simulink model "DDMR_sim_imputW"  (R2022a)
settings: Solver=FixedStepAuto  StartTime=0.0  StopTime=10.0  FixedStep=0.001  RelTol=1e-3
values from neighbouring files (symbols this model uses):
  Cm = 0    [DDMR_sim_imputW_set.m]
  Jm = 15.5*10^-7    (= 1.55e-06)    [DDMR_sim_imputW_set.m]
  Kb = Kt    (= 0.0286)    [DDMR_sim_imputW_set.m]
  Kf = 0    [DDMR_sim_imputW_set.m]
  Kt = 28.6*10^-3    (= 0.0286)    [DDMR_sim_imputW_set.m]
  La = 0.39*10^-3    (= 0.00039)    [DDMR_sim_imputW_set.m]
  N = N_motor * N_wheel    (= 1400)    [DDMR_sim_imputW_set.m]
  Ra = 0.38    [DDMR_sim_imputW_set.m]
libraries: simulink x2
settings Model: Creator=CSPLAB  LastModifiedBy=CSPLAB
settings DataIOCC: ReturnWorkspaceOutputs=off

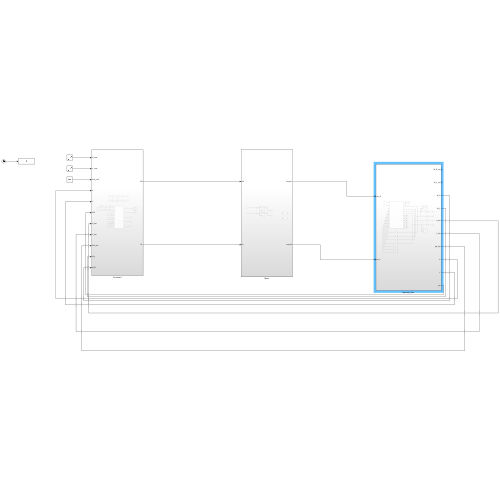
[thumbnail: Simulink's stored preview of the top-level diagram]
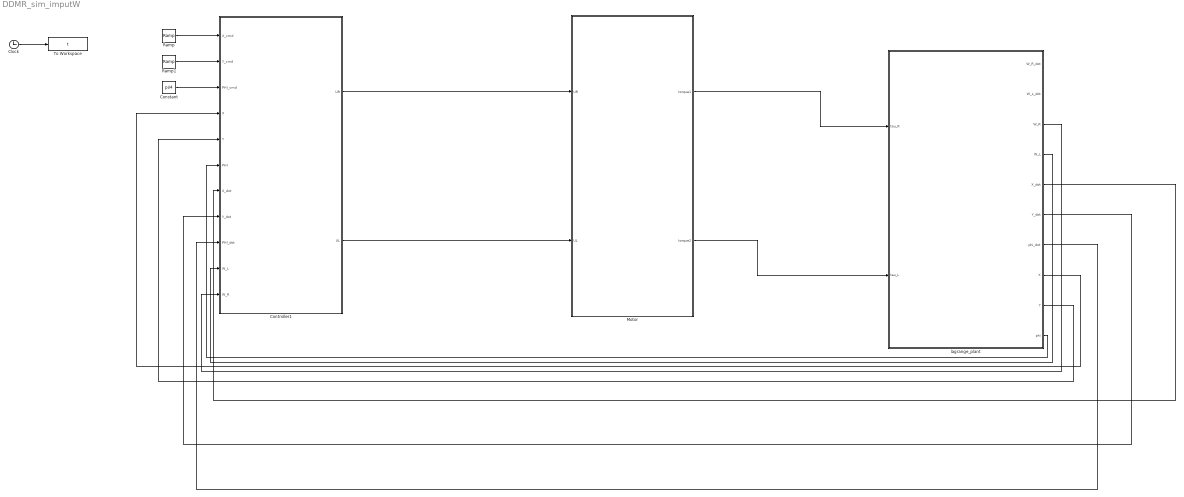
== system DDMR_sim_imputW ==
  Clock : Clock
  Constant : Constant  Value=pi/4
  Controller1 : Subsystem
  Motor : Subsystem
  Ramp : simulink/Sources/Ramp  slope=1  start=0  InitialOutput=0
  Ramp1 : simulink/Sources/Ramp  slope=1  start=0  InitialOutput=0
  To Workspace : ToWorkspace  VariableName=t  SaveFormat=Timeseries  SampleTime=-1
  lagrange_plant : Subsystem
  wires:
  Controller1/1(UR) -> Motor/1(UR)
  Controller1/2(UL) -> Motor/2(UL)
  Motor/1(torque1) -> lagrange_plant/1(tau_R)
  Motor/2(torque2) -> lagrange_plant/2(tau_L)
  lagrange_plant/3(W_R) -> Controller1/11(W_R)
  lagrange_plant/4(W_L) -> Controller1/10(W_L)
  Ramp1/1 -> Controller1/2(Y_cmd)
  Ramp/1 -> Controller1/1(X_cmd)
  Constant/1 -> Controller1/3(PHI_cmd)
  Clock/1 -> To Workspace/1
  lagrange_plant/10(phi) -> Controller1/6(PHI)
  lagrange_plant/5(X_dot) -> Controller1/7(X_dot)
  lagrange_plant/6(Y_dot) -> Controller1/8(Y_dot)
  lagrange_plant/7(phi_dot) -> Controller1/9(PHI_dot)
  lagrange_plant/8(X) -> Controller1/4(X)
  lagrange_plant/9(Y) -> Controller1/5(Y)

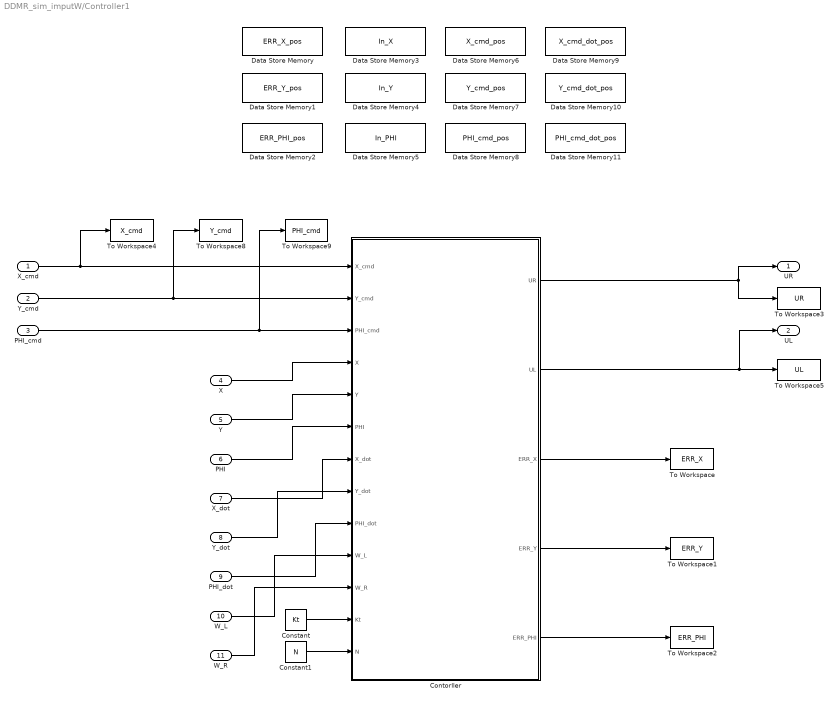
== system DDMR_sim_imputW/Controller1 ==
  X_cmd : Inport
  Y_cmd : Inport  Port=2
  PHI_cmd : Inport  Port=3
  X : Inport  Port=4
  Y : Inport  Port=5
  PHI : Inport  Port=6
  X_dot : Inport  Port=7
  Y_dot : Inport  Port=8
  PHI_dot : Inport  Port=9
  W_L : Inport  Port=10
  W_R : Inport  Port=11
  Constant : Constant  Value=Kt
  Constant1 : Constant  Value=N
  "Contorller " : MATLAB Function  TreatAsAtomicUnit=on
  Data Store Memory : DataStoreMemory  DataStoreName=ERR_X_pos  ReadBeforeWriteMsg=warning  WriteAfterWriteMsg=warning  WriteAfterReadMsg=warning  ShowAdditionalParam=off  OutDataTypeStr=double
  Data Store Memory1 : DataStoreMemory  DataStoreName=ERR_Y_pos  ReadBeforeWriteMsg=warning  WriteAfterWriteMsg=warning  WriteAfterReadMsg=warning  ShowAdditionalParam=off  OutDataTypeStr=double
  Data Store Memory10 : DataStoreMemory  DataStoreName=Y_cmd_dot_pos  ReadBeforeWriteMsg=warning  WriteAfterWriteMsg=warning  WriteAfterReadMsg=warning  ShowAdditionalParam=off  OutDataTypeStr=double
  Data Store Memory11 : DataStoreMemory  DataStoreName=PHI_cmd_dot_pos  ReadBeforeWriteMsg=warning  WriteAfterWriteMsg=warning  WriteAfterReadMsg=warning  ShowAdditionalParam=off  OutDataTypeStr=double
  Data Store Memory2 : DataStoreMemory  DataStoreName=ERR_PHI_pos  ReadBeforeWriteMsg=warning  WriteAfterWriteMsg=warning  WriteAfterReadMsg=warning  ShowAdditionalParam=off  OutDataTypeStr=double
  Data Store Memory3 : DataStoreMemory  DataStoreName=In_X  ReadBeforeWriteMsg=warning  WriteAfterWriteMsg=warning  WriteAfterReadMsg=warning  ShowAdditionalParam=off  OutDataTypeStr=double
  Data Store Memory4 : DataStoreMemory  DataStoreName=In_Y  ReadBeforeWriteMsg=warning  WriteAfterWriteMsg=warning  WriteAfterReadMsg=warning  ShowAdditionalParam=off  OutDataTypeStr=double
  Data Store Memory5 : DataStoreMemory  DataStoreName=In_PHI  ReadBeforeWriteMsg=warning  WriteAfterWriteMsg=warning  WriteAfterReadMsg=warning  ShowAdditionalParam=off  OutDataTypeStr=double
  Data Store Memory6 : DataStoreMemory  DataStoreName=X_cmd_pos  ReadBeforeWriteMsg=warning  WriteAfterWriteMsg=warning  WriteAfterReadMsg=warning  ShowAdditionalParam=off  OutDataTypeStr=double
  Data Store Memory7 : DataStoreMemory  DataStoreName=Y_cmd_pos  ReadBeforeWriteMsg=warning  WriteAfterWriteMsg=warning  WriteAfterReadMsg=warning  ShowAdditionalParam=off  OutDataTypeStr=double
  Data Store Memory8 : DataStoreMemory  DataStoreName=PHI_cmd_pos  ReadBeforeWriteMsg=warning  WriteAfterWriteMsg=warning  WriteAfterReadMsg=warning  ShowAdditionalParam=off  OutDataTypeStr=double
  Data Store Memory9 : DataStoreMemory  DataStoreName=X_cmd_dot_pos  ReadBeforeWriteMsg=warning  WriteAfterWriteMsg=warning  WriteAfterReadMsg=warning  ShowAdditionalParam=off  OutDataTypeStr=double
  To Workspace : ToWorkspace  VariableName=ERR_X  SampleTime=-1
  To Workspace1 : ToWorkspace  VariableName=ERR_Y  SampleTime=-1
  To Workspace2 : ToWorkspace  VariableName=ERR_PHI  SampleTime=-1
  To Workspace3 : ToWorkspace  VariableName=UR  SampleTime=-1
  To Workspace4 : ToWorkspace  VariableName=X_cmd  SampleTime=-1
  To Workspace5 : ToWorkspace  VariableName=UL  SampleTime=-1
  To Workspace8 : ToWorkspace  VariableName=Y_cmd  SampleTime=-1
  To Workspace9 : ToWorkspace  VariableName=PHI_cmd  SampleTime=-1
  UR : Outport  VectorParamsAs1DForOutWhenUnconnected=off
  UL : Outport  Port=2  VectorParamsAs1DForOutWhenUnconnected=off
  wires:
  "Contorller "/2(UL) -> UL/1, To Workspace5/1
  "Contorller "/1(UR) -> UR/1, To Workspace3/1
  W_R/1 -> "Contorller "/11(W_R)
  W_L/1 -> "Contorller "/10(W_L)
  PHI_dot/1 -> "Contorller "/9(PHI_dot)
  Y_dot/1 -> "Contorller "/8(Y_dot)
  X_dot/1 -> "Contorller "/7(X_dot)
  PHI/1 -> "Contorller "/6(PHI)
  Y/1 -> "Contorller "/5(Y)
  X/1 -> "Contorller "/4(X)
  PHI_cmd/1 -> To Workspace9/1, "Contorller "/3(PHI_cmd)
  Y_cmd/1 -> To Workspace8/1, "Contorller "/2(Y_cmd)
  X_cmd/1 -> To Workspace4/1, "Contorller "/1(X_cmd)
  Constant/1 -> "Contorller "/12(Kt)
  Constant1/1 -> "Contorller "/13(N)
  "Contorller "/5(ERR_PHI) -> To Workspace2/1
  "Contorller "/4(ERR_Y) -> To Workspace1/1
  "Contorller "/3(ERR_X) -> To Workspace/1

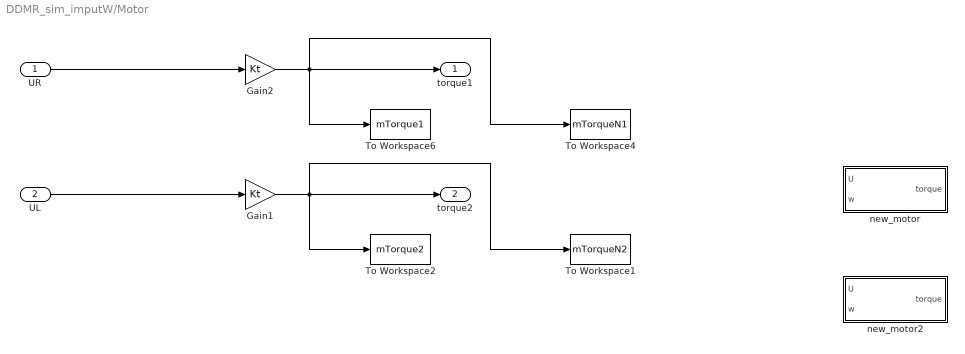
== system DDMR_sim_imputW/Motor ==
  UR : Inport
  UL : Inport  Port=2
  Gain1 : Gain  Gain=Kt
  Gain2 : Gain  Gain=Kt
  To Workspace1 : ToWorkspace  VariableName=mTorqueN2  SampleTime=-1
  To Workspace2 : ToWorkspace  VariableName=mTorque2  SampleTime=-1
  To Workspace4 : ToWorkspace  VariableName=mTorqueN1  SampleTime=-1
  To Workspace6 : ToWorkspace  VariableName=mTorque1  SampleTime=-1
  new_motor : Subsystem
  new_motor2 : Subsystem
  torque1 : Outport  VectorParamsAs1DForOutWhenUnconnected=off
  torque2 : Outport  Port=2  VectorParamsAs1DForOutWhenUnconnected=off
  wires:
  UR/1 -> Gain2/1
  Gain2/1 -> To Workspace6/1, To Workspace4/1, torque1/1
  Gain1/1 -> To Workspace2/1, To Workspace1/1, torque2/1
  UL/1 -> Gain1/1

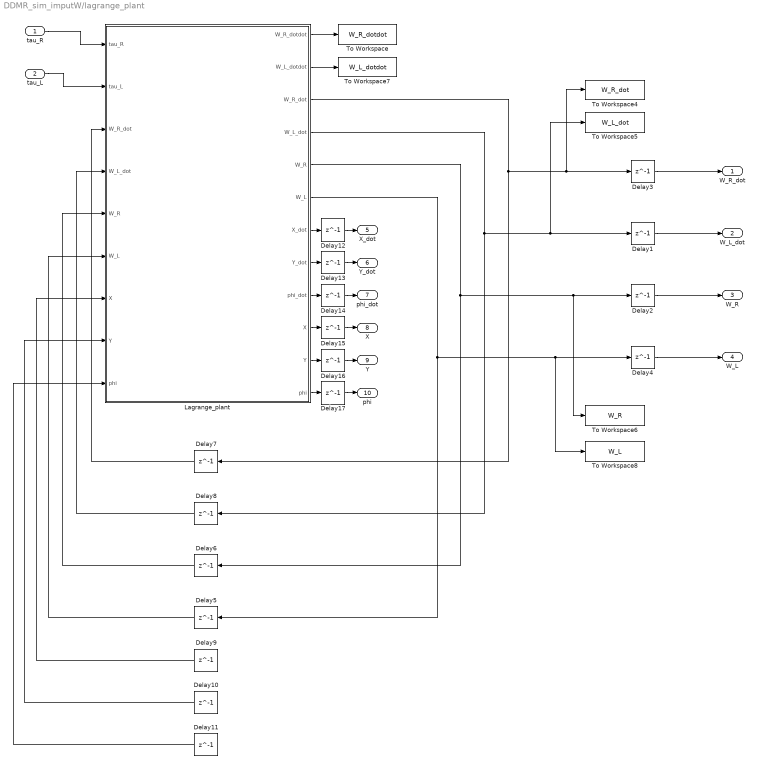
== system DDMR_sim_imputW/lagrange_plant ==
  tau_R : Inport
  tau_L : Inport  Port=2
  Delay{1..17} (17 alike) : Delay  DelayLength=1  InitialCondition=0
  Lagrange_plant : MATLAB Function  TreatAsAtomicUnit=on
  To Workspace : ToWorkspace  VariableName=W_R_dotdot  SaveFormat=Timeseries  SampleTime=-1
  To Workspace4 : ToWorkspace  VariableName=W_R_dot  SaveFormat=Timeseries  SampleTime=-1
  To Workspace5 : ToWorkspace  VariableName=W_L_dot  SaveFormat=Timeseries  SampleTime=-1
  To Workspace6 : ToWorkspace  VariableName=W_R  SaveFormat=Timeseries  SampleTime=-1
  To Workspace7 : ToWorkspace  VariableName=W_L_dotdot  SaveFormat=Timeseries  SampleTime=-1
  To Workspace8 : ToWorkspace  VariableName=W_L  SaveFormat=Timeseries  SampleTime=-1
  W_R_dot : Outport
  W_L_dot : Outport  Port=2
  W_R : Outport  Port=3
  W_L : Outport  Port=4
  X_dot : Outport  Port=5
  Y_dot : Outport  Port=6
  phi_dot : Outport  Port=7
  X : Outport  Port=8
  Y : Outport  Port=9
  phi : Outport  Port=10
  wires:
  Lagrange_plant/1(W_R_dotdot) -> To Workspace/1
  Lagrange_plant/2(W_L_dotdot) -> To Workspace7/1
  Delay1/1 -> W_L_dot/1
  Delay3/1 -> W_R_dot/1
  Delay2/1 -> W_R/1
  Delay4/1 -> W_L/1
  Lagrange_plant/6(W_L) -> Delay5/1, To Workspace8/1, Delay4/1
  Lagrange_plant/5(W_R) -> Delay6/1, To Workspace6/1, Delay2/1
  Lagrange_plant/4(W_L_dot) -> Delay8/1, Delay1/1, To Workspace5/1
  Lagrange_plant/3(W_R_dot) -> Delay7/1, To Workspace4/1, Delay3/1
  Delay7/1 -> Lagrange_plant/3("W_R_dot ")
  Delay8/1 -> Lagrange_plant/4("W_L_dot ")
  Delay6/1 -> Lagrange_plant/5("W_R ")
  Delay5/1 -> Lagrange_plant/6("W_L ")
  tau_R/1 -> Lagrange_plant/1(tau_R)
  tau_L/1 -> Lagrange_plant/2(tau_L)
  Delay9/1 -> Lagrange_plant/7("X ")
  Delay10/1 -> Lagrange_plant/8("Y ")
  Delay11/1 -> Lagrange_plant/9("phi ")
  Lagrange_plant/7(X_dot) -> Delay12/1
  Delay12/1 -> X_dot/1
  Lagrange_plant/8(Y_dot) -> Delay13/1
  Delay13/1 -> Y_dot/1
  Lagrange_plant/9(phi_dot) -> Delay14/1
  Delay14/1 -> phi_dot/1
  Lagrange_plant/10(X) -> Delay15/1
  Delay15/1 -> X/1
  Lagrange_plant/11(Y) -> Delay16/1
  Delay16/1 -> Y/1
  Lagrange_plant/12(phi) -> Delay17/1
  Delay17/1 -> phi/1

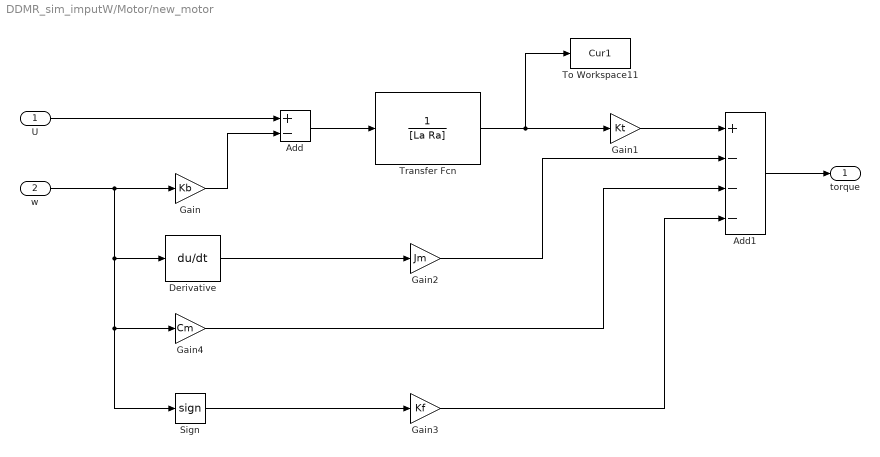
== system DDMR_sim_imputW/Motor/new_motor ==
  U : Inport
  w : Inport  Port=2
  Add : Sum  Inputs=+-
  Add1 : Sum  Inputs=+---
  Derivative : Derivative
  Gain : Gain  Gain=Kb
  Gain1 : Gain  Gain=Kt
  Gain2 : Gain  Gain=Jm
  Gain3 : Gain  Gain=Kf
  Gain4 : Gain  Gain=Cm
  Sign : Signum  ZeroCross=off
  To Workspace11 : ToWorkspace  VariableName=Cur1  SampleTime=-1
  Transfer Fcn : TransferFcn  Denominator=[La Ra]
  torque : Outport  VectorParamsAs1DForOutWhenUnconnected=off
  wires:
  Add1/1 -> torque/1
  Gain2/1 -> Add1/2
  Derivative/1 -> Gain2/1
  Gain1/1 -> Add1/1
  Gain4/1 -> Add1/3
  Gain/1 -> Add/2
  Transfer Fcn/1 -> To Workspace11/1, Gain1/1
  Sign/1 -> Gain3/1
  w/1 -> Sign/1, Gain4/1, Derivative/1, Gain/1
  U/1 -> Add/1
  Gain3/1 -> Add1/4
  Add/1 -> Transfer Fcn/1

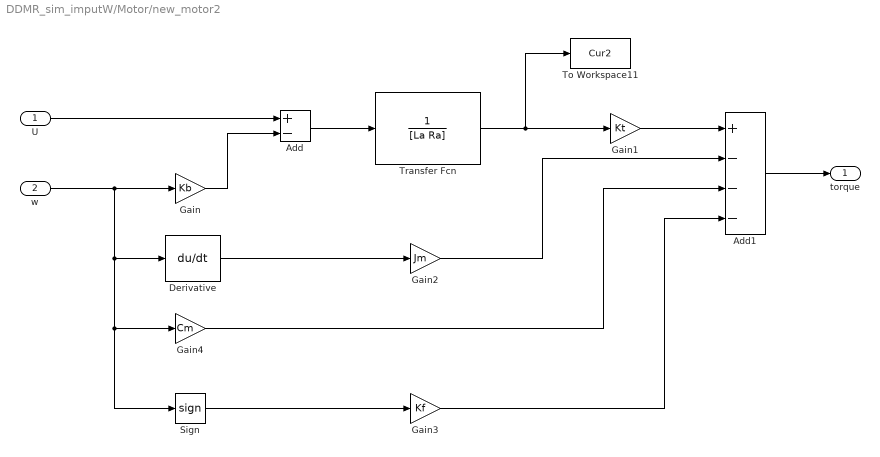
== system DDMR_sim_imputW/Motor/new_motor2 ==
  U : Inport
  w : Inport  Port=2
  Add : Sum  Inputs=+-
  Add1 : Sum  Inputs=+---
  Derivative : Derivative
  Gain : Gain  Gain=Kb
  Gain1 : Gain  Gain=Kt
  Gain2 : Gain  Gain=Jm
  Gain3 : Gain  Gain=Kf
  Gain4 : Gain  Gain=Cm
  Sign : Signum  ZeroCross=off
  To Workspace11 : ToWorkspace  VariableName=Cur2  SampleTime=-1
  Transfer Fcn : TransferFcn  Denominator=[La Ra]
  torque : Outport  VectorParamsAs1DForOutWhenUnconnected=off
  wires:
  Add1/1 -> torque/1
  Gain2/1 -> Add1/2
  Derivative/1 -> Gain2/1
  Gain1/1 -> Add1/1
  Gain4/1 -> Add1/3
  Add/1 -> Transfer Fcn/1
  Gain/1 -> Add/2
  Transfer Fcn/1 -> To Workspace11/1, Gain1/1
  Sign/1 -> Gain3/1
  w/1 -> Sign/1, Gain4/1, Derivative/1, Gain/1
  U/1 -> Add/1
  Gain3/1 -> Add1/4

== matlab function DDMR_sim_imputW/lagrange_plant/Lagrange_plant ==
  data: tau_R input; W_R_dotdot output; tau_L input; W_R_dot input; W_L_dot input; W_R input; W_L input; X input; Y input; phi input; W_L_dotdot output; W_R_dot output; W_L_dot output; W_R output; W_L output; X_dot output; Y_dot output; phi_dot output; X output; Y output; phi output
function [W_R_dotdot,W_L_dotdot,W_R_dot,W_L_dot,W_R,W_L,X_dot,Y_dot,phi_dot,X,Y,phi] = fcn(tau_R,tau_L,W_R_dot,W_L_dot,W_R,W_L,X,Y,phi)
%#codegen

%%
%parameter
dt = 0.001;

%car parameter
%重量單位:kg 
%長度單位:m

%body
m_b = 1200; 
d_b = 0.81;
L_b = 1.069; 
I_zb = 1/12*m_b*(d_b^2+L_b^2);
%wheel
m_w = 10; 
R = 0.09;
L = 0.4;
I_yw = m_w*R^2/2;
d = 0;
I_zw = m_w*(L^2 + d^2);


%dynamic model
BUFF = R^2/L^2*(I_zb+2*I_zw) + R^2/2*(m_b+2*m_w);

W_R_dotdot = (I_yw+BUFF)/(I_yw^2+2*BUFF*I_yw)*tau_R -(BUFF)/(I_yw^2+2*BUFF*I_yw)*tau_L;
W_L_dotdot = (I_yw+BUFF)/(I_yw^2+2*BUFF*I_yw)*tau_L -(BUFF)/(I_yw^2+2*BUFF*I_yw)*tau_R;

W_R_dot = W_R_dot + W_R_dotdot * dt;
W_L_dot = W_L_dot + W_L_dotdot * dt;

W_R = W_R + W_R_dot * dt;
W_L = W_L + W_L_dot * dt;

phi_dot =R/L*(W_R_dot - W_L_dot);
phi = phi + phi_dot*dt;

X_dot = (W_R_dot+W_L_dot)*R/2*cos(phi);
Y_dot = (W_R_dot+W_L_dot)*R/2*sin(phi);

X = X + X_dot*dt;
Y = Y + Y_dot*dt;

== matlab function DDMR_sim_imputW/Controller1/Contorller  ==
  settings: updateMethod=DISCRETE  sampleTime=0.001
  data: X_cmd input; UR output; UL output; Y_cmd input; PHI_cmd input; X input; Y input; PHI input; X_dot input; Y_dot input; PHI_dot input; W_L input; W_R input; ERR_X_pos data_store_memory; ERR_Y_pos data_store_memory; ERR_PHI_pos data_store_memory; In_X data_store_memory; In_Y data_store_memory; In_PHI data_store_memory; X_cmd_pos data_store_memory; Y_cmd_pos data_store_memory; PHI_cmd_pos data_store_memory; X_cmd_dot_pos data_store_memory; Y_cmd_dot_pos data_store_memory; PHI_cmd_dot_pos data_store_memory; ERR_X output; ERR_Y output; ERR_PHI output; Kt input; N input
function [UR,UL,ERR_X,ERR_Y,ERR_PHI]  = fcn(X_cmd,Y_cmd,PHI_cmd,X,Y,PHI,X_dot,Y_dot,PHI_dot,W_L,W_R,Kt,N)
%#codegen

global In_X
global In_Y
global In_PHI
global ERR_X_pos
global ERR_Y_pos
global ERR_PHI_pos
global X_cmd_pos
global Y_cmd_pos
global PHI_cmd_pos
global X_cmd_dot_pos
global Y_cmd_dot_pos
global PHI_cmd_dot_pos


%parameter
dt = 0.001;

%car parameter
%重量單位:kg 
%長度單位:m

%body
m_b = 1200; 
d_b = 0.81;
L_b = 1.069; 
I_zb = 1/12*m_b*(d_b^2+L_b^2);
%wheel
m_w = 10; 
R = 0.09;
L = 0.4;
I_yw = m_w*R^2/2;
d = 0;
I_zw = m_w*(L^2 + d^2);

% %=== Motor ===
% Ra = 0.38;
% Kt = 28.6*10^-3;
% Kb = Kt;
% 
% %=== Gear ===
% N = 14;

%=== Sat ===
MaxU = 24;

dt = 0.001;


%===== Controller =====
Kp = 10;
Ki = 0;
Kd = 0;

ERR_X   = X_cmd   - X;
ERR_Y   = Y_cmd   - Y;
ERR_PHI = PHI_cmd - PHI;



% ===== X =====
X_cmd_dot = (X_cmd - X_cmd_pos)/dt ;
X_cmd_dotdot = (X_cmd_dot - X_cmd_dot_pos)/dt;

Pr_X = Kp*ERR_X;
In_X = In_X + Ki*ERR_X*dt;
Di_X = Kd*(ERR_X-ERR_X_pos)/dt;

X_all =  X_cmd_dotdot + Pr_X + In_X + Di_X ;

% ===== Y =====
Y_cmd_dot = (Y_cmd - Y_cmd_pos)*dt ;
Y_cmd_dotdot = (Y_cmd_dot - Y_cmd_dot_pos)*dt;

Pr_Y = Kp*ERR_Y;
In_Y = In_Y + Ki*ERR_Y*dt;
Di_Y = Kd*(ERR_Y-ERR_Y_pos)/dt;

Y_all = Y_cmd_dotdot + Pr_Y + In_Y + Di_Y ;

% ===== PHI =====
PHI_cmd_dot = (PHI_cmd - PHI_cmd_pos)/dt ;
PHI_cmd_dotdot = (PHI_cmd_dot - PHI_cmd_dot_pos)/dt;

Pr_PHI = Kp*ERR_PHI;
In_PHI = In_PHI + Ki*ERR_PHI*dt;
Di_PHI = Kd*(ERR_PHI-ERR_PHI_pos)/dt;

PHI_all = PHI_cmd_dotdot + Pr_PHI + In_PHI + Di_PHI;


% ===== TQC =====
BUFF_POSI = 2*I_yw*+R^2*m_b+2*R^2*m_w;
BUFF_ANGLE = -I_yw*L^2+2*I_zb*R^2+4*I_zw*R^2+L^2*R^2*m_w;

% === MR ====
Buff_X   =  sin(PHI)/(2*R)*BUFF_POSI;
Buff_Y   =  cos(PHI)/(2*R)*BUFF_POSI;
Buff_PHI =  -BUFF_ANGLE/(2*L*R);

TQC1 = (Buff_X*X_all + Buff_Y*Y_all + Buff_PHI*PHI_all)/N;

% === ML ====
Buff_X   =  sin(PHI)/(2*R)*BUFF_POSI;
Buff_Y   =  cos(PHI)/(2*R)*BUFF_POSI;
Buff_PHI =  BUFF_ANGLE/(2*L*R);

TQC2 = (Buff_X*X_all + Buff_Y*Y_all + Buff_PHI*PHI_all)/N;




% TQC_to_Uc

UR = TQC1/Kt;
UL = TQC2/Kt;


if ( abs(UR)>MaxU )
    UR =sign(UR)*MaxU;
end

if ( abs(UL)>MaxU )
    UL =sign(UL)*MaxU;
end





%===== Recorder =====
X_cmd_pos = X_cmd;
Y_cmd_pos = Y_cmd;
PHI_cmd_pos = PHI_cmd;

X_cmd_dot_pos = X_cmd_dot;
Y_cmd_dot_pos = Y_cmd_dot;
PHI_cmd_dot_pos = PHI_cmd_dot;

ERR_X_pos   = ERR_X;
ERR_Y_pos   = ERR_Y;
ERR_PHI_pos = ERR_PHI;
